simulink model "DT_DSM_CRFF_LOWPASS_2nd_2048"  (R2025b)
settings: Solver=VariableStepAuto  StartTime=0.0  StopTime=1  RelTol=1e-3
libraries: simulink_extras x1
settings Model: Creator=Team_33  LastModifiedBy=k2vas

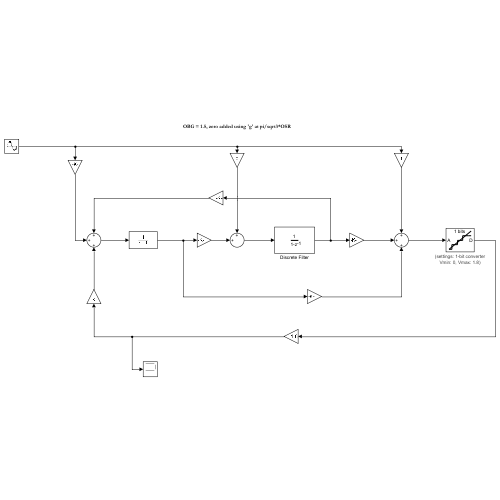
[thumbnail: Simulink's stored preview of the top-level diagram]
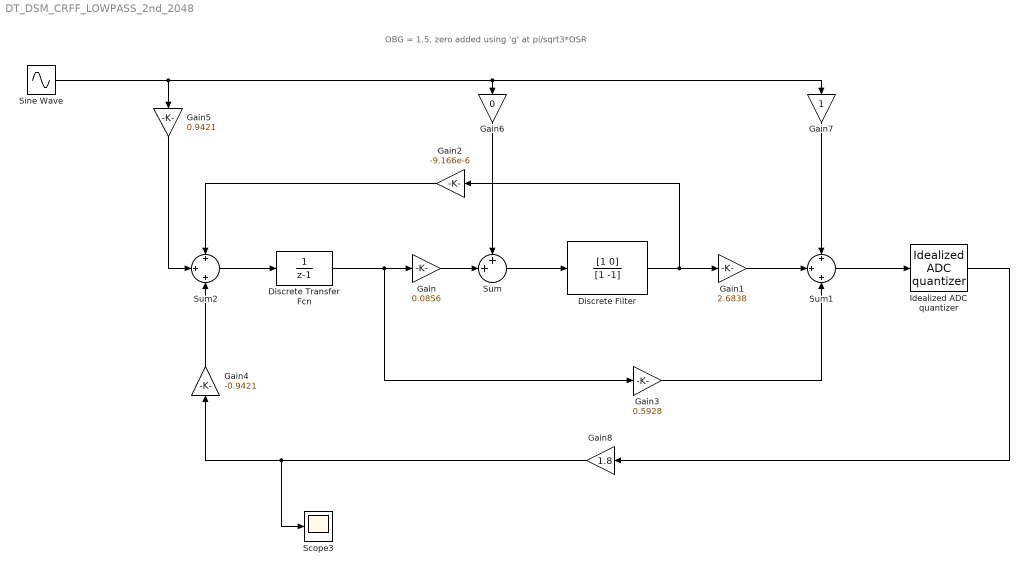
== system DT_DSM_CRFF_LOWPASS_2nd_2048 ==
  note: OBG = 1.5, zero added using 'g' at pi/sqrt3*OSR
  Discrete Transfer Fcn : DiscreteTransferFcn  Denominator=[1 -1]
  Discrete Filter : DiscreteFilter  Numerator=[1 0]  Denominator=[1 -1]  InputProcessing=Columns as channels (frame based)  FilterStructure=Direct form II transposed  a0EqualsOne=on
  Gain : Gain  Gain=0.0856
  Gain1 : Gain  Gain=2.6838
  Gain2 : Gain  Gain=-9.166e-6
  Gain3 : Gain  Gain=0.5928
  Gain4 : Gain  Gain=-0.9421
  Gain5 : Gain  Gain=0.9421
  Gain6 : Gain  Gain=0
  Gain7 : Gain
  Gain8 : Gain  Gain=1.8
  Idealized ADC quantizer : simulink_extras/Additional Discrete/Idealized ADC quantizer  NumberOfConverterBits=1  Vmin=0  Vmax=1.8  OutputDataType=int16  OutputNegativeValues=off
  Scope3 : Scope
      settings: ActiveDisplayYMinimum=1.03994  ActiveDisplayYMaximum=1.04051  DataLoggingVariableName=output_data  DataLoggingSaveFormat=Array
  Sine Wave : Sin  Amplitude=0.6  Bias=0.9  Frequency=(2000*2048)*(2*pi*127)/(32768*32)  SampleTime=1/(2000*2048)
  Sum : Sum  Inputs=++|
  Sum1 : Sum  Inputs=+|+|+
  Sum2 : Sum  Inputs=+|+|+
  wires:
  Discrete Transfer Fcn/1 -> Gain3/1, Gain/1
  Discrete Filter/1 -> Gain2/1, Gain1/1
  Gain/1 -> Sum/2
  Sum/1 -> Discrete Filter/1
  Gain1/1 -> Sum1/2
  Sum1/1 -> Idealized ADC quantizer/1
  Sum2/1 -> Discrete Transfer Fcn/1
  Gain2/1 -> Sum2/1
  Gain3/1 -> Sum1/3
  Idealized ADC quantizer/1 -> Gain8/1
  Gain4/1 -> Sum2/3
  Gain7/1 -> Sum1/1
  Gain6/1 -> Sum/1
  Gain5/1 -> Sum2/2
  Sine Wave/1 -> Gain7/1, Gain6/1, Gain5/1
  Gain8/1 -> Scope3/1, Gain4/1
